simulink model "rel2"  (Simulink 7.1)
settings: Solver=ode45  StartTime=0.0  StopTime=10.0  RelTol=1e-3
settings Model: Creator=Erica 8D  LastModifiedBy=Erica 8D

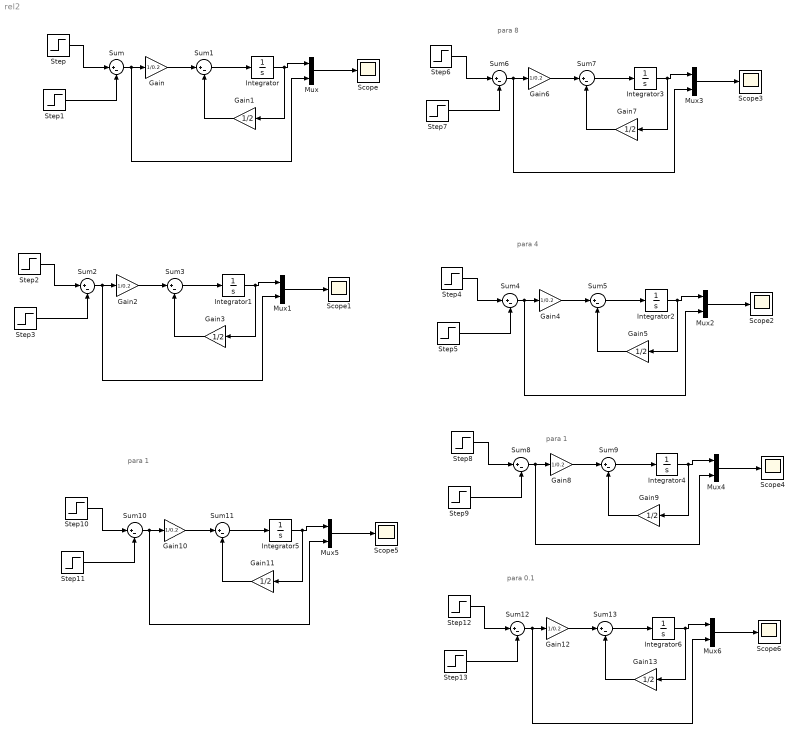
== system rel2 ==
  note: para 0.1
  note: para 1
  note: para 1
  note: para 4
  note: para 8
  Gain{,2,4,6,8,10,12} (7 alike) : Gain  Gain=1/0.2  ParameterDataType=sfix(16)  ParameterScaling=2^0  OutDataType=sfix(16)  OutScaling=2^0
  Gain{1,3,5,7,9,11,13} (7 alike) : Gain  Orientation=left  Gain=1/2  ParameterDataType=sfix(16)  ParameterScaling=2^0  OutDataType=sfix(16)  OutScaling=2^0
  Integrator{,1..6} (7 alike) : Integrator
  Mux{,1..6} (7 alike) : Mux  Inputs=2
  Scope{,1..6} (7 alike) : Scope
      Scope2 settings: SaveName=ScopeData2
      Scope3 settings: SaveName=ScopeData3
      Scope4 settings: SaveName=ScopeData4
      Scope5 settings: SaveName=ScopeData5
      Scope6 settings: SaveName=ScopeData6
  Step{,2,4,6,8,10,12} (7 alike) : Step  SampleTime=0
  Step1 : Step  Time=2  SampleTime=0
  Step11 : Step  Time=2  SampleTime=0
  Step13 : Step  Time=1.1  SampleTime=0
  Step3 : Step  Time=0  After=0  SampleTime=0
  Step5 : Step  Time=5  SampleTime=0
  Step7 : Step  Time=9  SampleTime=0
  Step9 : Step  Time=2  SampleTime=0
  Sum{,1..13} (14 alike) : Sum  Inputs=|+-  OutDataType=sfix(16)  OutScaling=2^0
  wires:
  Step/1 -> Sum/1
  Step1/1 -> Sum/2
  Sum/1 -> Gain/1, Mux/2
  Gain/1 -> Sum1/1
  Gain1/1 -> Sum1/2
  Sum1/1 -> Integrator/1
  Integrator/1 -> Mux/1, Gain1/1
  Mux/1 -> Scope/1
  Step2/1 -> Sum2/1
  Step3/1 -> Sum2/2
  Sum2/1 -> Gain2/1, Mux1/2
  Gain2/1 -> Sum3/1
  Gain3/1 -> Sum3/2
  Sum3/1 -> Integrator1/1
  Integrator1/1 -> Mux1/1, Gain3/1
  Mux1/1 -> Scope1/1
  Step6/1 -> Sum6/1
  Step7/1 -> Sum6/2
  Sum6/1 -> Gain6/1, Mux3/2
  Gain6/1 -> Sum7/1
  Gain7/1 -> Sum7/2
  Sum7/1 -> Integrator3/1
  Integrator3/1 -> Mux3/1, Gain7/1
  Mux3/1 -> Scope3/1
  Step4/1 -> Sum4/1
  Step5/1 -> Sum4/2
  Sum4/1 -> Gain4/1, Mux2/2
  Gain4/1 -> Sum5/1
  Gain5/1 -> Sum5/2
  Sum5/1 -> Integrator2/1
  Integrator2/1 -> Mux2/1, Gain5/1
  Mux2/1 -> Scope2/1
  Step8/1 -> Sum8/1
  Step9/1 -> Sum8/2
  Sum8/1 -> Gain8/1, Mux4/2
  Gain8/1 -> Sum9/1
  Gain9/1 -> Sum9/2
  Sum9/1 -> Integrator4/1
  Integrator4/1 -> Mux4/1, Gain9/1
  Mux4/1 -> Scope4/1
  Step10/1 -> Sum10/1
  Step11/1 -> Sum10/2
  Sum10/1 -> Gain10/1, Mux5/2
  Gain10/1 -> Sum11/1
  Gain11/1 -> Sum11/2
  Sum11/1 -> Integrator5/1
  Integrator5/1 -> Mux5/1, Gain11/1
  Mux5/1 -> Scope5/1
  Step12/1 -> Sum12/1
  Step13/1 -> Sum12/2
  Sum12/1 -> Gain12/1, Mux6/2
  Gain12/1 -> Sum13/1
  Gain13/1 -> Sum13/2
  Sum13/1 -> Integrator6/1
  Integrator6/1 -> Mux6/1, Gain13/1
  Mux6/1 -> Scope6/1
